simulink model "Gamepad_Xbox_test_drive"  (R2026a)
settings: Solver=VariableStepAuto  StopTime=inf
undefined symbols (not defined in the file): Driver
libraries: Gamepad_Xbox x1
Description:
  | Copyright 2020-2026 The MathWorks, Inc.
settings Model: Creator=smiller  LastModifiedBy=smiller

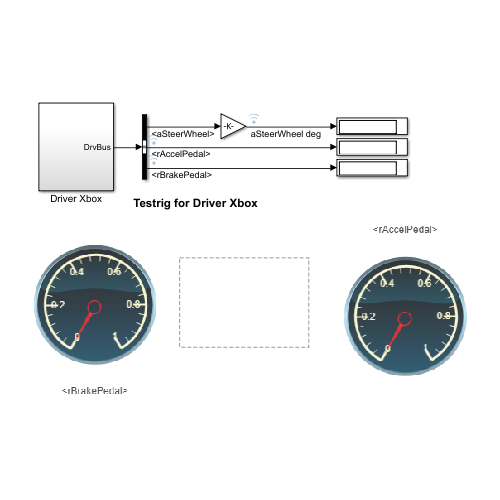
[thumbnail: Simulink's stored preview of the top-level diagram]
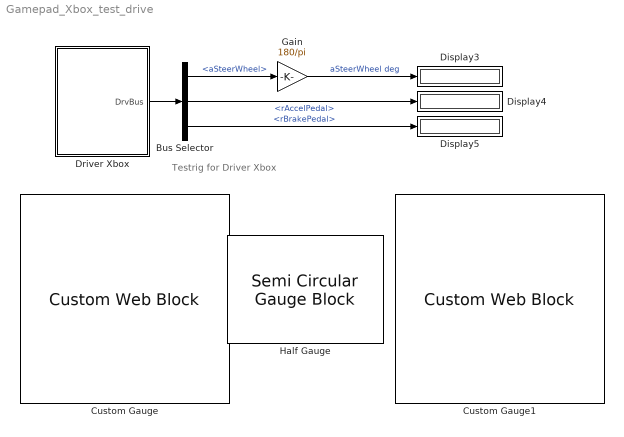
== system Gamepad_Xbox_test_drive ==
  note: Testrig for Driver Xbox
  Bus Selector : BusSelector  OutputSignals=aSteerWheel,rAccelPedal,rBrakePedal
  Custom Gauge : CustomWebBlock  LabelPosition=Bottom  ShowInitialText=on  Configuration="{\"components\":[{\"name\":\"CircularScaleComponent\",\"settings\":{\"bounds\":{\"max\":1,\"min\":0,\"tickInterval\":\"auto\"},\"direction\":\"cw\",\"flipLimits\":0,\"innerRadius\":0.5279616348635409,\"internalTickHeightScaleFactor\":1,\"labelColor\":[250,245,200],\"labelFont\":{\"font\":\"Arial\",\"fontSize\":12},\"labelRadius\":0.528,\"labelTransparency\":1,\"labelTrasparency\":1,\"minorTickHeightScaleFactor\":0.2,\"needleImage\":{\"size\":[1890,567],\"src\":\"data:image\\/svg+xml;base64,PD94bWwgdmVyc2lvbj0iMS4wIiBlbmNvZGluZz0iVVRGLTgiIHN0YW5kYWxvbmU9Im5vIj8+CjxzdmcKICAgeG1sbnM6ZGM9Imh0dHA6Ly9wdXJsLm9yZy9kYy9lbGVtZW50cy8xLjEvIgogICB4bWxuczpjYz0iaHR0cDovL2NyZWF0aXZlY29tbW9ucy5vcmcvbnMjIgogICB4bWxuczpyZGY9Imh0dHA6Ly93d3cudzMub3JnLzE5OTkvMDIvMjItcmRmLXN5bnRheC1ucyMiCiAgIHhtbG5zOnN2Zz0iaHR0cDovL3d3dy53My5vcmcvMjAwMC9zdmciCiAgIHhtbG5zPSJodHRwOi8vd3d3LnczLm9yZy8yMDAwL3N2ZyIKICAgeG1sbnM6 ...(+4096 chars)\"},\"needleOffset\":[0.1275,0],\"needleOrientation\":-45,\"needleRotation\":180,\"needleSize\":{\"height\":0.1036,\"width\":0.3364},\"outerRadius\":0.7088000664454559,\"position\":[0.06486742424242424,0.05627705627705628,0.8917748917748918,0.8787878787878788],\"referencePoint\":\"auto\",\"scaleAngle\":299.999999999988,\"scaleAngleOffset\":119.46147497096791,\"scaleColors\":[],\"scaleColorsSize\":0.2,\"scaleDirection\":\"CW\",\"scalePosition\":[0,0,1,1],\"showLabels\":1,\"showMinorTicks\":1,\"showSpanLine\":1,\"showTicks\":1,\"tickColor\":[250,245,200],\"tickTransparency\":1,\"valueBarColor\":[23,89,176],\"valueBarPosition\":[0,0,1,1],\"valueBarSize\":0.2,\"valueBarTransparency\":1}},{\"name\":\"BackgroundImageComponent\",\"settings\":{\"image\":{\"size\":[500,500],\"src\":\"data:image\\/svg+xml;base64,PD94bWwgdmVyc2lvbj0iMS4wIiBlbmNvZGluZz0iVVRGLTgiIHN0YW5kYWxvbmU9Im5vIj8+CjwhLS0gR2VuZXJhdG9yOiBBZG9iZSBJbGx1c3RyYXRvciAxOS4yLjEsIFNWRyBFeHBvcnQgUGx1Zy1JbiAuIFNWRyBWZXJzaW9uOiA2LjAwIEJ1aWxkIDApICAtLT4KCjxzdmcKICAgeG1sbnM6ZGM9Imh0dHA6Ly9wdXJsLm9yZy9kYy9lbGVtZW50cy8xLjEvIgogICB4bWxuczpjYz0iaHR0cDovL2NyZWF0aXZlY29tbW9ucy5vcmcvbnMjIgogICB4bWxuczpyZGY9Imh0dHA6Ly93d3cudzMub3JnLzE5OTkvMDIvMjItcmRmLXN5bnRh ...(+9660 chars)\",\"srcOrientation\":\"horizontal\"},\"position\":[0,0,1,1],\"scaleMode\":\"0\"}},{\"name\":\"ForegroundImageComponent\",\"settings\":{\"image\":{\"size\":[0,0],\"src\":\"default\",\"srcOrientation\":[]},\"isForeground\":1,\"position\":[0,0,1,1],\"scaleMode\":\"0\"}}],\"derived\":{\"blockParameters\":{\"ForegroundColor\":[0.9803921568627451,0.9607843137254902,0.7843137254901961],\"Limits\":{\"Max\":1,\"Min\":0,\"Ticks\":\"auto\"},\"ScaleColors\":[],\"ScaleDirection\":\"Clockwise\",\"ScaleMax\":1,\"ScaleMin\":0,\"TickInterval\":\"auto\",\"fixedAspectRatio\":\"on\"}},\"settings\":{\"BindingType\":\"signal\",\"aspectRatio\":1,\"backgroundOffset\":0.14,\"fixedAspectRatio\":\"on\",\"orientation\":\"horizontal\",\"version\":\"R2022b\"},\"type\":\"CircularGauge\"}"
  Custom Gauge1 : CustomWebBlock  ShowInitialText=on  Configuration="{\"components\":[{\"name\":\"CircularScaleComponent\",\"settings\":{\"bounds\":{\"max\":1,\"min\":0,\"tickInterval\":\"auto\"},\"direction\":\"cw\",\"flipLimits\":0,\"innerRadius\":0.5279616348635409,\"internalTickHeightScaleFactor\":1,\"labelColor\":[250,245,200],\"labelFont\":{\"font\":\"Arial\",\"fontSize\":12},\"labelRadius\":0.528,\"labelTransparency\":1,\"labelTrasparency\":1,\"minorTickHeightScaleFactor\":0.2,\"needleImage\":{\"size\":[1890,567],\"src\":\"data:image\\/svg+xml;base64,PD94bWwgdmVyc2lvbj0iMS4wIiBlbmNvZGluZz0iVVRGLTgiIHN0YW5kYWxvbmU9Im5vIj8+CjxzdmcKICAgeG1sbnM6ZGM9Imh0dHA6Ly9wdXJsLm9yZy9kYy9lbGVtZW50cy8xLjEvIgogICB4bWxuczpjYz0iaHR0cDovL2NyZWF0aXZlY29tbW9ucy5vcmcvbnMjIgogICB4bWxuczpyZGY9Imh0dHA6Ly93d3cudzMub3JnLzE5OTkvMDIvMjItcmRmLXN5bnRheC1ucyMiCiAgIHhtbG5zOnN2Zz0iaHR0cDovL3d3dy53My5vcmcvMjAwMC9zdmciCiAgIHhtbG5zPSJodHRwOi8vd3d3LnczLm9yZy8yMDAwL3N2ZyIKICAgeG1sbnM6 ...(+4096 chars)\"},\"needleOffset\":[0.1275,0],\"needleOrientation\":-45,\"needleRotation\":180,\"needleSize\":{\"height\":0.1036,\"width\":0.3364},\"outerRadius\":0.7088000664454559,\"position\":[0.06486742424242424,0.05627705627705628,0.8917748917748918,0.8787878787878788],\"referencePoint\":\"auto\",\"scaleAngle\":299.999999999988,\"scaleAngleOffset\":119.46147497096791,\"scaleColors\":[],\"scaleColorsSize\":0.2,\"scaleDirection\":\"CW\",\"scalePosition\":[0,0,1,1],\"showLabels\":1,\"showMinorTicks\":1,\"showSpanLine\":1,\"showTicks\":1,\"tickColor\":[250,245,200],\"tickTransparency\":1,\"valueBarColor\":[23,89,176],\"valueBarPosition\":[0,0,1,1],\"valueBarSize\":0.2,\"valueBarTransparency\":1}},{\"name\":\"BackgroundImageComponent\",\"settings\":{\"image\":{\"size\":[500,500],\"src\":\"data:image\\/svg+xml;base64,PD94bWwgdmVyc2lvbj0iMS4wIiBlbmNvZGluZz0iVVRGLTgiIHN0YW5kYWxvbmU9Im5vIj8+CjwhLS0gR2VuZXJhdG9yOiBBZG9iZSBJbGx1c3RyYXRvciAxOS4yLjEsIFNWRyBFeHBvcnQgUGx1Zy1JbiAuIFNWRyBWZXJzaW9uOiA2LjAwIEJ1aWxkIDApICAtLT4KCjxzdmcKICAgeG1sbnM6ZGM9Imh0dHA6Ly9wdXJsLm9yZy9kYy9lbGVtZW50cy8xLjEvIgogICB4bWxuczpjYz0iaHR0cDovL2NyZWF0aXZlY29tbW9ucy5vcmcvbnMjIgogICB4bWxuczpyZGY9Imh0dHA6Ly93d3cudzMub3JnLzE5OTkvMDIvMjItcmRmLXN5bnRh ...(+9660 chars)\",\"srcOrientation\":\"horizontal\"},\"position\":[0,0,1,1],\"scaleMode\":\"0\"}},{\"name\":\"ForegroundImageComponent\",\"settings\":{\"image\":{\"size\":[0,0],\"src\":\"default\",\"srcOrientation\":[]},\"isForeground\":1,\"position\":[0,0,1,1],\"scaleMode\":\"0\"}}],\"derived\":{\"blockParameters\":{\"ForegroundColor\":[0.9803921568627451,0.9607843137254902,0.7843137254901961],\"Limits\":{\"Max\":1,\"Min\":0,\"Ticks\":\"auto\"},\"ScaleColors\":[],\"ScaleDirection\":\"Clockwise\",\"ScaleMax\":1,\"ScaleMin\":0,\"TickInterval\":\"auto\",\"fixedAspectRatio\":\"on\"}},\"settings\":{\"BindingType\":\"signal\",\"aspectRatio\":1,\"backgroundOffset\":0.14,\"fixedAspectRatio\":\"on\",\"orientation\":\"horizontal\",\"version\":\"R2022b\"},\"type\":\"CircularGauge\"}"
  Display3 : Display
  Display4 : Display
  Display5 : Display
  Driver Xbox : Subsystem
  Gain : Gain  Gain=180/pi
  Half Gauge : SemiCircularGaugeBlock  ScaleMin=-80  ScaleMax=80  FontColor=[0.0, 0.0, 0.0]
  wires:
  Driver Xbox/1(DrvBus) -> Bus Selector/1
  Bus Selector/1 -> Gain/1  "<aSteerWheel>"
  Bus Selector/2 -> Display4/1  "<rAccelPedal>"
  Bus Selector/3 -> Display5/1  "<rBrakePedal>"
  Gain/1 -> Display3/1  "aSteerWheel deg"

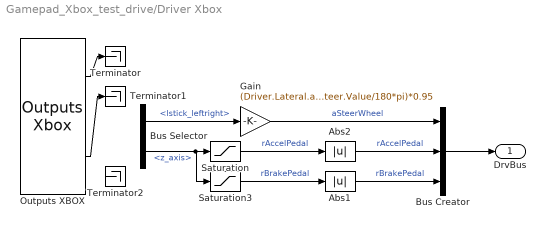
== system Gamepad_Xbox_test_drive/Driver Xbox ==
  Abs1 : Abs  ZeroCross=off  SaturateOnIntegerOverflow=off
  Abs2 : Abs  ZeroCross=off  SaturateOnIntegerOverflow=off
  Bus Creator : BusCreator  Inputs=3
  Bus Selector : BusSelector  OutputSignals=lstick_leftright,z_axis
  Gain : Gain  Gain=(Driver.Lateral.aMaxSteer.Value/180*pi)*0.95
  Outputs XBOX : Gamepad_Xbox/Outputs Xbox  DLx=0.07  DLy=0.05  Dz=0.01  DRx=0.04  DRy=0.01  joyid=1
  Saturation : Saturate  UpperLimit=0  LowerLimit=-1  ZeroCross=off
  Saturation3 : Saturate  UpperLimit=1  LowerLimit=0  ZeroCross=off
  Terminator : Terminator
  Terminator1 : Terminator
  Terminator2 : Terminator
  DrvBus : Outport  VectorParamsAs1DForOutWhenUnconnected=off
  wires:
  Saturation/1 -> Abs2/1  "rAccelPedal"
  Bus Selector/2 -> Saturation3/1, Saturation/1  "<z_axis>"
  Saturation3/1 -> Abs1/1  "rBrakePedal"
  Outputs XBOX/1 -> Terminator/1
  Outputs XBOX/2 -> Terminator1/1
  Abs1/1 -> Bus Creator/3  "rBrakePedal"
  ? -> Bus Selector/1
  ? -> Terminator2/1
  Abs2/1 -> Bus Creator/2  "rAccelPedal"
  Gain/1 -> Bus Creator/1  "aSteerWheel"
  Bus Selector/1 -> Gain/1  "<lstick_leftright>"
  Bus Creator/1 -> DrvBus/1
